simulink model "environment_test"  (R2016b)
settings: Solver=VariableStepAuto  StartTime=0.0  StopTime=5400  RelTol=1e-3
libraries: dynamics_lib x1, environment_lib x1
settings Model: Creator=taylorreynolds  LastModifiedBy=taylorreynolds

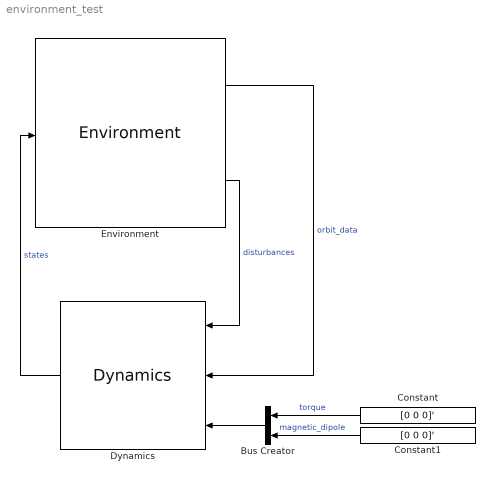
== system environment_test ==
  Bus Creator : BusCreator  Inputs=2
  Constant : Constant  Value=[0 0 0]'
  Constant1 : Constant  Value=[0 0 0]'
  Dynamics : dynamics_lib/Dynamics
  Environment : environment_lib/Environment
  wires:
  Environment/1 -> Dynamics/2  "orbit_data"
  Environment/2 -> Dynamics/1  "disturbances"
  Bus Creator/1 -> Dynamics/3
  Dynamics/1 -> Environment/1  "states"
  Constant/1 -> Bus Creator/1  "torque"
  Constant1/1 -> Bus Creator/2  "magnetic_dipole"
